simulink model "current_ctl_tf_sim"  (R2023a)
settings: configuration reference "config" (kept outside this file)
model workspace (MATLAB code in the model file + MAT data in the model file):
  cmdLim = Simulink.Parameter
  cmdLim.Value = 15
  cmdLim.Description = 'Limit for controlling the maximum surface command angle.'
  cmdLim.Min = 0
  cmdLim.Max = 90
  cmdLim.DocUnits = 'deg'
  dispGain = Simulink.Parameter
  dispGain.Value = 0.75
  dispGain.Description = 'Gain applied to the displacement error.'
  dispGain.Min = 0
  dispGain.Max = []
  dispGain.DocUnits = 'deg/sec/deg'
  dispLim = Simulink.Parameter
  dispLim.Value = 30
  dispLim.Description = 'Limit for controlling the maximum commanded angle.'
  dispLim.Min = 0
  dispLim.Max = 180
  dispLim.DocUnits = 'deg'
  intGain = Simulink.Parameter
  intGain.Value = 0.5
  intGain.Description = 'Gain applied to the integral error.'
  intGain.Min = 0
  intGain.Max = []
  intGain.DocUnits = 'deg/sec/deg/sec'
  intLim = Simulink.Parameter
  intLim.Value = 5
  intLim.Description = 'Limit for controlling the maximum commanded angle.'
  intLim.Min = 0
  intLim.Max = 90
  intLim.DocUnits = 'deg'
  rateGain = Simulink.Parameter
  rateGain.Value = 2
  rateGain.Description = 'Gain applied to the rate error.'
  rateGain.Min = 0
  rateGain.Max = []
  rateGain.DocUnits = 'deg/deg/sec'
  rateLim = Simulink.Parameter
  rateLim.Value = 6
  rateLim.Description = 'Limit for controlling the maximum commanded angle.'
  rateLim.Min = 0
  rateLim.Max = 180
  rateLim.DocUnits = 'deg/sec'
  hdgGain = Simulink.Parameter
  hdgGain.Value = 0.015
  J1 = Simulink.Parameter
  J1.Value = 1.1e-05
  J1.DataType = 'double'
  J1.Complexity = 'real'
  J1.Dimensions = [1 1]
  J2 = Simulink.Parameter
  J2.Value = 0.000208
  J2.DataType = 'double'
  J2.Complexity = 'real'
  J2.Dimensions = [1 1]
  K = Simulink.Parameter
  K.Value = 20
  K.DataType = 'double'
  K.Complexity = 'real'
  K.Dimensions = [1 1]
  b = Simulink.Parameter
  b.Value = 0.001
  b.DataType = 'single'
  b.Complexity = 'real'
  b.Dimensions = [1 1]
  current_ctl_bw_rad_s = Simulink.Parameter
  current_ctl_bw_rad_s.Value = 6666.7
  current_ctl_bw_rad_s.Description = '电流环设计带宽'
  current_ctl_bw_rad_s.DataType = 'single'
  current_ctl_bw_rad_s.Complexity = 'real'
  current_ctl_bw_rad_s.Dimensions = [1 1]
  dt = Simulink.Parameter
  dt.Value = 1e-05
  dt.DataType = 'single'
  dt.Complexity = 'real'
  dt.Dimensions = [1 1]
  enc_line = Simulink.Parameter
  enc_line.Value = 10000
  enc_line.Description = '编码器分辨率 脉冲每圈'
  enc_line.DataType = 'single'
  enc_line.Complexity = 'real'
  enc_line.Dimensions = [1 1]
  fc = Simulink.Parameter
  fc.Value = 0.001
  fc.DataType = 'single'
  fc.Complexity = 'real'
  fc.Dimensions = [1 1]
  flux = Simulink.Parameter
  flux.Value = 0.0083
  flux.DataType = 'single'
  flux.Complexity = 'real'
  flux.Dimensions = [1 1]
  fs = Simulink.Parameter
  fs.Value = 10000
  fs.Description = '位置环 速度环执行频率'
  fs.DataType = 'single'
  fs.Complexity = 'real'
  fs.Dimensions = [1 1]
  j = Simulink.Parameter
  j.Value = 1.9e-05
  j.DataType = 'single'
  j.Complexity = 'real'
  j.Dimensions = [1 1]
  j_inv = Simulink.Parameter
  j_inv.Value = 100000
  j_inv.DataType = 'single'
  j_inv.Complexity = 'real'
  j_inv.Dimensions = [1 1]
  kt = Simulink.Parameter
  kt.Value = 0.075
  kt.DataType = 'single'
  kt.Complexity = 'real'
  kt.Dimensions = [1 1]
  ld = Simulink.Parameter
  ld.Value = 0.00059
  ld.DataType = 'single'
  ld.Complexity = 'real'
  ld.Dimensions = [1 1]
  ld_inv = Simulink.Parameter
  ld_inv.Value = 1694.91525424
  ld_inv.DataType = 'single'
  ld_inv.Complexity = 'real'
  ld_inv.Dimensions = [1 1]
  lq = Simulink.Parameter
  lq.Value = 0.00059
  lq.DataType = 'single'
  lq.Complexity = 'real'
  lq.Dimensions = [1 1]
  lq_inv = Simulink.Parameter
  lq_inv.Value = 1694.91525424
  lq_inv.DataType = 'single'
  lq_inv.Complexity = 'real'
  lq_inv.Dimensions = [1 1]
  pn = Simulink.Parameter
  pn.Value = 4
  pn.DataType = 'single'
  pn.Complexity = 'real'
  pn.Dimensions = [1 1]
  r = Simulink.Parameter
  r.Value = 1.02
  r.DataType = 'single'
  r.Complexity = 'real'
  r.Dimensions = [1 1]
  tc = Simulink.Parameter
  tc.Value = 5e-05
  tc.Description = '电流环运行频率用来设定综合仿真的参数'
  tc.DataType = 'double'
  tc.Complexity = 'real'
  tc.Dimensions = [1 1]
  tp = Simulink.Parameter
  tp.Value = 0.0001
  tp.Description = '位置环速度环执行周期'
  tp.DataType = 'double'
  tp.Complexity = 'real'
  tp.Dimensions = [1 1]
  ts = Simulink.Parameter
  ts.Value = 1e-05
  ts.Description = '模型仿真的周期 s'
  ts.DataType = 'double'
  ts.Complexity = 'real'
  ts.Dimensions = [1 1]
undefined symbols (not defined in the file): DiscIntNeverNeededParam
libraries: dspsrcs4 x1
settings Model: RequirementInfo={} %GIDa_fe9045fd_0412_4b6e_8206_617cc20e6fde  DataDictionary=model_config.sldd  ParameterArgumentNames=J1,J2,K,b,current_ctl_bw_rad_s,dt,enc_line,fc,flux,fs,j,j_inv,kt,ld,ld_inv,lq,lq_inv,pn,r  Creator=Administrator  LastModifiedBy=Administrator
settings ConfigSetRef: SourceName=config

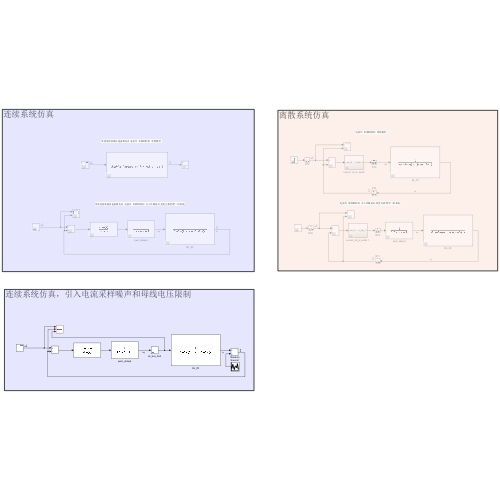
[thumbnail: Simulink's stored preview of the top-level diagram]
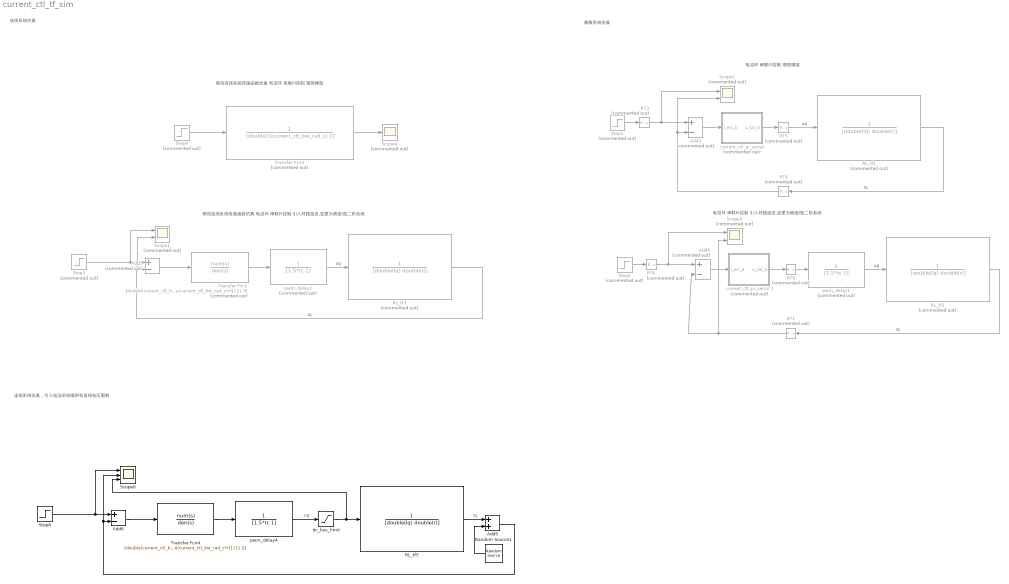
== system current_ctl_tf_sim ==
  note: 离散系统仿真
  note: 连续系统仿真
  note: 电流环 串联PI控制 理想模型
  note: 电流环 串联PI控制 引入环路延迟,变更为典型I型二阶系统
  note: 等效连续系统传递函数仿真 电流环 串联PI控制 理想模型
  note: 等效连续系统传递函数仿真 电流环 串联PI控制 引入环路延迟,变更为典型I型二阶系统
  note: 连续系统仿真，引入电流采样噪声和母线电压限制
  Add2 : Sum  Commented=on  Inputs=+-
  Add3 : Sum  Commented=on  Inputs=+-
  Add4 : Sum  Commented=on  Inputs=+-
  Add5 : Sum
  Add6 : Sum  Inputs=+-
  RL_tf1 : TransferFcn  Commented=on  Denominator=[double(lq) double(r)]
  RL_tf2 : TransferFcn  Commented=on  Denominator=[double(lq) double(r)]
  RL_tf3 : TransferFcn  Commented=on  Denominator=[double(lq) double(r)]
  RL_tf5 : TransferFcn  Denominator=[double(lq) double(r)]
  RT{1,3..4,6} (4 alike) : RateTransition  Commented=on  OutPortSampleTime=tc
  RT5 : RateTransition  Commented=on  OutPortSampleTime=1e-05
  RT8 : RateTransition  Commented=on  OutPortSampleTime=1e-05
  Random Source1 : dspsrcs4/Random Source  SrcType=Uniform  NormMethod=Ziggurat  CltLength=12  MinVal=-0.2  MaxVal=0.2  MeanVal=0  VarVal=1  RepMode=Not repeatable  rawSeed=1  IsInherit=off  SampMode=Discrete  SampTime=-1  SampFrame=1  DataType=Double  OutComplex=Real  OutputFrames=off
  Scope1 : Scope  Commented=on  NumInputPorts=2
  Scope2 : Scope  Commented=on  NumInputPorts=2
  Scope3 : Scope  Commented=on  NumInputPorts=2
  Scope4 : Scope  Commented=on
  Scope6 : Scope  NumInputPorts=3
  Step{1..4} (4 alike) : Step  Commented=on  SampleTime=0
  Step6 : Step  SampleTime=0
  Transfer Fcn2 : TransferFcn  Commented=on  Numerator=[double(current_ctl_bw_rad_s*lq) double(current_ctl_bw_rad_s*r)]  Denominator=[1 0]
  Transfer Fcn3 : TransferFcn  Commented=on  Denominator=[double(1/current_ctl_bw_rad_s) 1]
  Transfer Fcn4 : TransferFcn  Numerator=[double(current_ctl_bw_rad_s*lq) double(current_ctl_bw_rad_s*r)]  Denominator=[1 0]
  "current_ctl_pi_serial " : Subsystem  Commented=on
  current_ctl_pi_serial 1 : Subsystem  Commented=on
  dc_bus_limit : Saturate  UpperLimit=12  LowerLimit=-12
  pwm_delay1 : TransferFcn  Commented=on  Denominator=[1.5*tc 1]
  pwm_delay2 : TransferFcn  Commented=on  Denominator=[1.5*tc 1]
  pwm_delay4 : TransferFcn  Denominator=[1.5*tc 1]
  wires:
  Step1/1 -> RT3/1
  RT4/1 -> Add3/2, Scope2/2
  RT5/1 -> RL_tf1/1  "uq"
  RT3/1 -> Add3/1, Scope2/1
  "current_ctl_pi_serial "/1(u_tar_V) -> RT5/1
  RL_tf1/1 -> RT4/1  "iq"
  Add3/1 -> "current_ctl_pi_serial "/1(i_err_A)
  Add4/1 -> current_ctl_pi_serial 1/1(i_err_A)
  RL_tf2/1 -> RT1/1  "iq"
  current_ctl_pi_serial 1/1(u_tar_V) -> RT8/1
  RT6/1 -> Add4/1, Scope3/1
  RT8/1 -> pwm_delay1/1
  Step2/1 -> RT6/1
  pwm_delay1/1 -> RL_tf2/1  "uq"
  RT1/1 -> Scope3/2, Add4/2
  Step4/1 -> Transfer Fcn3/1
  Transfer Fcn3/1 -> Scope4/1
  Add2/1 -> Transfer Fcn2/1
  Step3/1 -> Scope1/1, Add2/1
  Transfer Fcn2/1 -> pwm_delay2/1
  RL_tf3/1 -> Scope1/2, Add2/2  "iq"
  pwm_delay2/1 -> RL_tf3/1  "uq"
  Add6/1 -> Transfer Fcn4/1
  Step6/1 -> Scope6/1, Add6/1
  pwm_delay4/1 -> dc_bus_limit/1  "uq"
  Transfer Fcn4/1 -> pwm_delay4/1
  dc_bus_limit/1 -> Scope6/3, RL_tf5/1
  RL_tf5/1 -> Add5/1  "iq"
  Random Source1/1 -> Add5/2
  Add5/1 -> Scope6/2, Add6/2

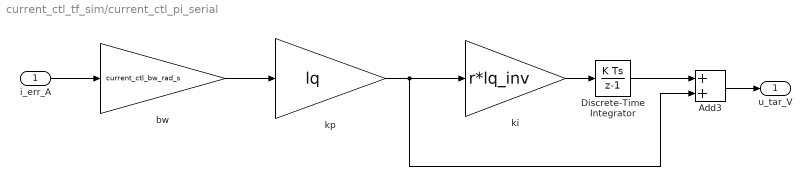
== system current_ctl_tf_sim/current_ctl_pi_serial  ==
  i_err_A : Inport
  Add3 : Sum
  Discrete-Time Integrator : DiscreteIntegrator  SampleTime=-1  ICPrevOutput=DiscIntNeverNeededParam  ICPrevScaledInput=DiscIntNeverNeededParam
  bw : Gain  Gain=current_ctl_bw_rad_s
  ki : Gain  Gain=r*lq_inv
  kp : Gain  Gain=lq
  u_tar_V : Outport
  wires:
  Add3/1 -> u_tar_V/1
  Discrete-Time Integrator/1 -> Add3/1
  i_err_A/1 -> bw/1
  ki/1 -> Discrete-Time Integrator/1
  kp/1 -> Add3/2, ki/1
  bw/1 -> kp/1

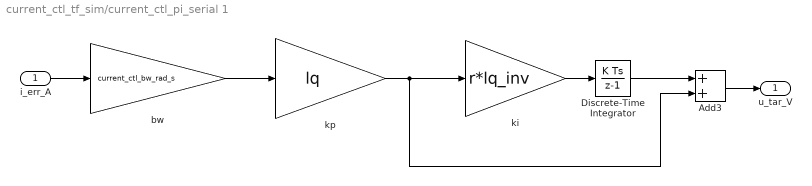
== system current_ctl_tf_sim/current_ctl_pi_serial 1 ==
  i_err_A : Inport
  Add3 : Sum
  Discrete-Time Integrator : DiscreteIntegrator  SampleTime=-1  ICPrevOutput=DiscIntNeverNeededParam  ICPrevScaledInput=DiscIntNeverNeededParam
  bw : Gain  Gain=current_ctl_bw_rad_s
  ki : Gain  Gain=r*lq_inv
  kp : Gain  Gain=lq
  u_tar_V : Outport
  wires:
  Add3/1 -> u_tar_V/1
  Discrete-Time Integrator/1 -> Add3/1
  i_err_A/1 -> bw/1
  ki/1 -> Discrete-Time Integrator/1
  kp/1 -> Add3/2, ki/1
  bw/1 -> kp/1
